simulink model "Torque_Control"  (R2022a)
settings: Solver=FixedStepAuto  StartTime=0.0  StopTime=10.0  RelTol=1e-3
libraries: simulink x9, eeGeneralControl x3
(part 1 of 6)
settings Model: Creator=cspt  LastModifiedBy=joser
settings SolverCC: AlgebraicLoopSolver=TrustRegion
settings DataIOCC: ReturnWorkspaceOutputs=off
settings DebuggingCC: UnconnectedInputMsg=warning  UnconnectedOutputMsg=warning  UnconnectedLineMsg=warning  ArithmeticOperatorsInVariantConditions=warning
settings SFSimCC: SimUseLocalCustomCode=off  CustomCodeUndefinedFunction=UseInterfaceOnly
settings RTWCC: Description=INTECRIO Real-Time Target  SystemTargetFile=irt.tlc  TemplateMakefile=irt_default_tmf  RTWUseLocalCustomCode=off
settings STFCustomTargetCC: TargetLangStandard=C99 (ISO)  UtilityFuncGeneration=Shared location  SystemTargetFile=irt.tlc
settings GRTTargetCC: UtilityFuncGeneration=Shared location  ParMdlRefBuildCompliant=off  CompOptLevelCompliant=off  ConcurrentExecutionCompliant=off  CombineOutputUpdateFcns=off  MatFileLogging=off  CPPClassGenCompliant=off  GRTInterface=on  UseToolchainInfoCompliant=off  GenerateASAP2=on

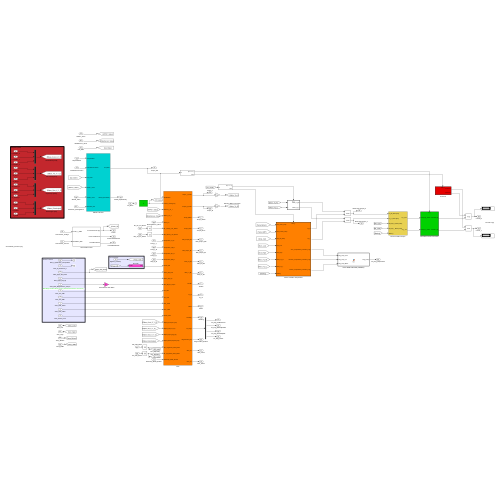
[thumbnail: Simulink's stored preview of the top-level diagram]
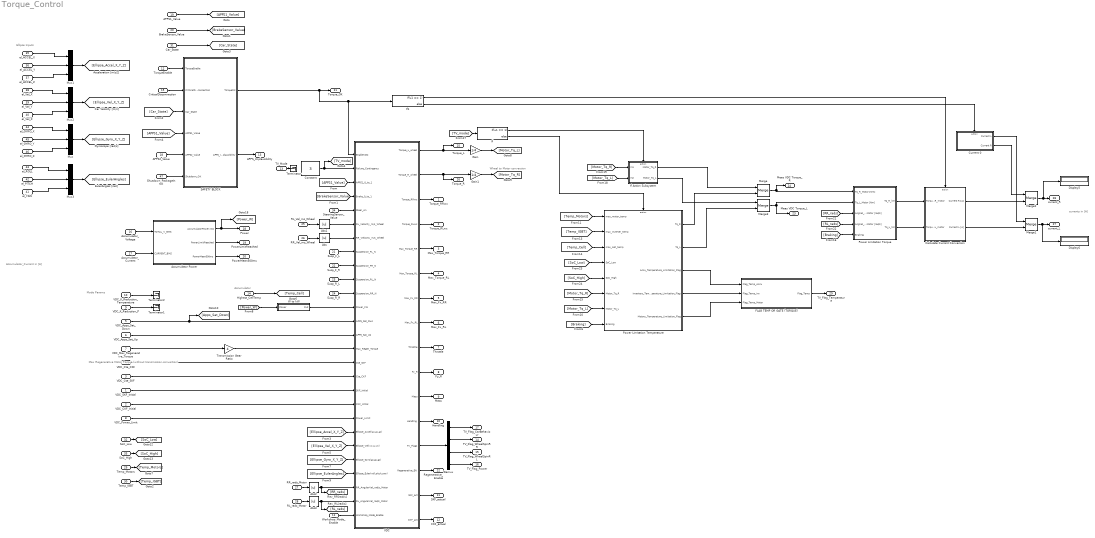
== system Torque_Control ==
  note: Ellipse Inputs
  note: Accumulator_Current in [A]
  note: Wheel to Motor conversion
  note: Max Regenerative Motor Torque (without transmission convertion)
  note: Mode Params
  note: Accumulator
  note: currents in [A]
  VDC_SKF_Initial : Inport
  VDC_CKF_Initial : Inport  Port=2
  VDC_Cte_SKF : Inport  Port=3
  VDC_Cte_CKF : Inport  Port=4
  VDC_Apps_Sat_Down : Inport  Port=5
  VDC_Apps_Sat_Up : Inport  Port=6
  VDC_Max_Regenerative_Torque : Inport  Port=7
  VDC_Power_Limit : Inport  Port=8
  VDC_K_Reduction_P : Inport  Port=9
  VDC_K_Reduction_Temperature : Inport  Port=10
  Workshop_Mode_Enable : Inport  Port=11
  TorqueEnable : Inport  Port=12
  TV_Mode : Inport  Port=13
  Highest_CellTemp : Inport  Port=14
  CriticalDisconnection : Inport  Port=15
  Accumulator_Voltage : Inport  Port=16
  Accumulator_Current : Inport  Port=17
  APPS2_Value : Inport  Port=18
  APPS1_Value : Inport  Port=19
  BrakeSensor_Value : Inport  Port=20
  Susp_F_L : Inport  Port=21
  Susp_F_R : Inport  Port=22
  Susp_R_L : Inport  Port=23
  Susp_R_R : Inport  Port=24
  RL_Vel_ms_Wheel : Inport  Port=25
  RR_Vel_ms_Wheel : Inport  Port=26
  RR_rads_Motor : Inport  Port=27
  RL_rads_Motor : Inport  Port=28
  Temp_Motors : Inport  Port=29
  Temp_IGBT : Inport  Port=30
  Car_State : Inport  Port=31
  SoC_Low : Inport  Port=32
  SoC_High : Inport  Port=33
  SteeringSensor_Value : Inport  Port=34
  el_ACCEL_X : Inport  Port=35
  el_ACCEL_Y : Inport  Port=36
  el_ACCEL_Z : Inport  Port=37
  el_Vel_X : Inport  Port=38
  el_Vel_Y : Inport  Port=39
  el_Vel_Z : Inport  Port=40
  el_YAW : Inport  Port=41
  el_PITCH : Inport  Port=42
  el_ROLL : Inport  Port=43
  el_GYRO_X : Inport  Port=44
  el_GYRO_Y : Inport  Port=45
  el_GYRO_Z : Inport  Port=46
  Shutdown_PackageIntck : Inport  Port=47
  Abs{,1..3} (4 alike) : Abs  SaturateOnIntegerOverflow=off
  Accumulator Power : Subsystem
  Calculate Current Conversion : Subsystem
  Constant : Constant  Value=3
  Current 0 : Subsystem  TreatAsAtomicUnit=on
  Demux : Demux
  Display5 : Display
  Display6 : Display
  FLAG TEMP OR GATE (TORQUE) : MATLAB Function  TreatAsAtomicUnit=on
  Gain : Gain  Gain=1/4
  Gain1 : Gain  Gain=1/4
  If : If  IfExpression=u1 == 1
  If Action Subsystem : Subsystem  TreatAsAtomicUnit=on
  If1 : If  IfExpression=u1 == 1
  Merge{,1..3} (4 alike) : Merge
  Mux{,1..3} (4 alike) : Mux  Inputs=3
  Power Limitation Temperature : Subsystem  TreatAsAtomicUnit=on
  Power Limitation Torque : Subsystem
  SAFETY BLOCK : Subsystem
  Terminator : Terminator
  Terminator1 : Terminator
  Terminator2 : Terminator
  Transmission Gear Ratio : Gain  Gain=4
  VDC : Subsystem
  W to kW : Subsystem
  Torque_RRwc : Outport  VectorParamsAs1DForOutWhenUnconnected=off
  Torque_RLwc : Outport  Port=2  VectorParamsAs1DForOutWhenUnconnected=off
  Max_Torque_RR : Outport  Port=3  VectorParamsAs1DForOutWhenUnconnected=off
  Max_Torque_RL : Outport  Port=4  VectorParamsAs1DForOutWhenUnconnected=off
  Max_Fx_RR : Outport  Port=5  VectorParamsAs1DForOutWhenUnconnected=off
  Max_Fx_RL : Outport  Port=6  VectorParamsAs1DForOutWhenUnconnected=off
  Throttle : Outport  Port=7  VectorParamsAs1DForOutWhenUnconnected=off
  Fy_R : Outport  Port=8  VectorParamsAs1DForOutWhenUnconnected=off
  Mass : Outport  Port=9  VectorParamsAs1DForOutWhenUnconnected=off
  Handling : Outport  Port=10  VectorParamsAs1DForOutWhenUnconnected=off
  SKF_actual : Outport  Port=11  VectorParamsAs1DForOutWhenUnconnected=off
  CKF_actual : Outport  Port=12  VectorParamsAs1DForOutWhenUnconnected=off
  APPS_Implausibility : Outport  Port=13  VectorParamsAs1DForOutWhenUnconnected=off
  TV_Flag_WheelSpinRR : Outport  Port=14  VectorParamsAs1DForOutWhenUnconnected=off
  TV_Flag_WheelSpinRL : Outport  Port=15  VectorParamsAs1DForOutWhenUnconnected=off
  TV_Flag_Power : Outport  Port=16  VectorParamsAs1DForOutWhenUnconnected=off
  TV_Flag_CarBehaviour : Outport  Port=17  VectorParamsAs1DForOutWhenUnconnected=off
  Power : Outport  Port=18  VectorParamsAs1DForOutWhenUnconnected=off
  PowerLimitReached : Outport  Port=19  VectorParamsAs1DForOutWhenUnconnected=off
  PowerMean500ms : Outport  Port=20  VectorParamsAs1DForOutWhenUnconnected=off
  Torque_OK : Outport  Port=21  VectorParamsAs1DForOutWhenUnconnected=off
  Regenerative_Enable : Outport  Port=22  VectorParamsAs1DForOutWhenUnconnected=off
  Meas VDC Torque_L : Outport  Port=23  VectorParamsAs1DForOutWhenUnconnected=off
  Meas VDC Torque_R : Outport  Port=24  VectorParamsAs1DForOutWhenUnconnected=off
  Torque_L : Outport  Port=25  VectorParamsAs1DForOutWhenUnconnected=off
  Torque_R : Outport  Port=26  VectorParamsAs1DForOutWhenUnconnected=off
  current_L : Outport  Port=27  VectorParamsAs1DForOutWhenUnconnected=off
  current_R : Outport  Port=28  VectorParamsAs1DForOutWhenUnconnected=off
  TV_Flag_Temperature : Outport  Port=29  VectorParamsAs1DForOutWhenUnconnected=off
  wires:
  Accumulator Power/1(AccumulatorPower [W]) -> [Power_W], Power/1
  Workshop_Mode_Enable/1 -> VDC/27(Workshop_Mode_Enable)
  SAFETY BLOCK/2(APPS_Implausibility) -> APPS_Implausibility/1
  VDC_Cte_SKF/1 -> VDC/17(Cte_CKF)
  VDC_Apps_Sat_Down/1 -> [Apps_Sat_Down], VDC/13(APPS_Sat_Dwn)
  VDC_Cte_CKF/1 -> VDC/16(Cte_SKF)
  VDC_SKF_Initial/1 -> VDC/18(SKF_Initial)
  VDC/3(Torque_RRwc) -> Torque_RRwc/1
  Highest_CellTemp/1 -> [Temp_Cell]
  [Car_State] -> SAFETY BLOCK/3(Car_State)
  Accumulator_Current/1 -> Accumulator Power/2(CURRENT_BMS)
  Accumulator Power/3(PowerMean500ms) -> PowerMean500ms/1
  Demux/1 -> TV_Flag_CarBehaviour/1
  VDC/14(Regenerative_EN) -> Regenerative_Enable/1
  VDC/10(Fy_R) -> Fy_R/1
  If1/2 -> Current 0/Action
  If1/1 -> Calculate Current Conversion/Action
  TorqueEnable/1 -> SAFETY BLOCK/1(TorqueEnable)
  VDC/5(Max_Torque_RR) -> Max_Torque_RR/1
  Accumulator_Voltage/1 -> Accumulator Power/1(TOTAL_V_BMS)
  Accumulator Power/2(PowerLimitReached) -> PowerLimitReached/1
  VDC/7(Max_Fx_RR) -> Max_Fx_RR/1
  VDC/8(Max_Fx_RL) -> Max_Fx_RL/1
  VDC_CKF_Initial/1 -> VDC/19(CKF_Initial)
  Demux/2 -> TV_Flag_WheelSpinRR/1
  VDC/9(Throttle) -> Throttle/1
  Demux/3 -> TV_Flag_WheelSpinRL/1
  [Power_W] -> W to kW/1(Power)
  CriticalDisconnection/1 -> SAFETY BLOCK/2(CriticalDisconnection)
  VDC/11(Mass) -> Mass/1
  VDC/16(CKF_act) -> CKF_actual/1
  VDC/12(Handling) -> Handling/1
  VDC/13(TV_Flags) -> Demux/1
  VDC/6(Max_Torque_RL) -> Max_Torque_RL/1
  VDC/15(SKF_act) -> SKF_actual/1
  VDC/4(Torque_RLwc) -> Torque_RLwc/1
  APPS1_Value/1 -> [APPS1_Value]
  BrakeSensor_Value/1 -> [BrakeSensor_Value]
  Susp_F_L/1 -> VDC/8(Suspension_FL_N)
  Susp_F_R/1 -> VDC/9(Suspension_FR_N)
  Susp_R_L/1 -> VDC/10(Suspension_RL_N)
  Susp_R_R/1 -> VDC/11(Suspension_RR_N)
  APPS2_Value/1 -> SAFETY BLOCK/5(APPS2_Value)
  Car_State/1 -> [Car_State]
  Abs/1 -> VDC/7(RR_Velocity_m/s_Wheel)
  Abs1/1 -> VDC/6(RL_Velocity_m/s_Wheel)
  Abs2/1 -> [RR_rads], VDC/25(RR_AngularVel_rad/s_Motor)
  Merge1/1 -> current_L/1, Display6/1
  Merge2/1 -> Display5/1, current_R/1
  W to kW/1(Out) -> VDC/12(Power_kW)
  VDC_K_Reduction_P/1 -> Terminator1/1
  VDC_K_Reduction_Temperature/1 -> Terminator2/1
  Demux/4 -> TV_Flag_Power/1
  Current 0/1(Current L) -> Merge1/1
  Transmission Gear Ratio/1 -> VDC/15(Max_Regen_Torque)
  Temp_Motors/1 -> [Temp_Motors]
  Temp_IGBT/1 -> [Temp_IGBT]
  VDC/1(Torque_L_wheel) -> Torque_L/1, Gain/1
  [APPS1_Value] -> VDC/3(APPS1_0_to_1)
  [BrakeSensor_Value] -> VDC/4(Brake_0_to_1)
  [Motor_Tq_R] -> Power Limitation Temperature/6(Motor_Tq_R)
  [Motor_Tq_L] -> Power Limitation Temperature/7(Motor_Tq_L)
  [Temp_Motors] -> Power Limitation Temperature/1(max_motor_temp)
  SoC_High/1 -> [SoC_High]
  [Temp_Cell] -> Power Limitation Temperature/3(max_cell_temp)
  Power Limitation Temperature/4(Inverters_Temperature_Limitation_Flag) -> FLAG TEMP OR GATE (TORQUE)/2(Flag_Temp_Inv)
  Power Limitation Temperature/3(Accu_Temperature_Limitation_Flag) -> FLAG TEMP OR GATE (TORQUE)/1(Flag_Temp_Accu)
  [TV_mode] -> If/1
  Gain1/1 -> [Motor_Tq_R]
  Gain/1 -> [Motor_Tq_L]
  Merge3/1 -> Power Limitation Torque/2(Tq_L_Motor [Nm]), Meas VDC Torque_L/1
  If/1 -> If Action Subsystem/Action
  [Motor_Tq_R] -> If Action Subsystem/1(In1)
  [Motor_Tq_L] -> If Action Subsystem/2(In2)
  Merge/1 -> Power Limitation Torque/1(Tq_R_Motor [Nm]), Meas VDC Torque_R/1
  If/2 -> Power Limitation Temperature/Action
  If Action Subsystem/1(Motor_Tq_R) -> Merge/1
  If Action Subsystem/2(Motor_Tq_L) -> Merge3/1
  Power Limitation Temperature/1(Tq_R) -> Merge/2
  Power Limitation Temperature/2(Tq_L) -> Merge3/2
  RL_Vel_ms_Wheel/1 -> Abs1/1
  RR_Vel_ms_Wheel/1 -> Abs/1
  RR_rads_Motor/1 -> Abs2/1
  RL_rads_Motor/1 -> Abs3/1
  VDC_Max_Regenerative_Torque/1 -> Transmission Gear Ratio/1
  SoC_Low/1 -> [SoC_Low]
  [Temp_IGBT] -> Power Limitation Temperature/2(max_inverter_temp)
  Power Limitation Temperature/5(Motors_Temperature_Limitation_Flag) -> FLAG TEMP OR GATE (TORQUE)/3(Flag_Temp_Motor)
  [Braking] -> Power Limitation Temperature/8(Braking)
  Current 0/2(Current R) -> Merge2/1
  SAFETY BLOCK/1(TorqueOK) -> Torque_OK/1, If1/1, VDC/1(EnableVDC)
  [RR_rads] -> Power Limitation Torque/3(AngVel_R_Motor [rad/s])
  [RL_rads] -> Power Limitation Torque/4(AngVel_L_Motor [rad/s])
  [Braking] -> Power Limitation Torque/5(Braking)
  Power Limitation Torque/1(Tq_R_lim) -> Calculate Current Conversion/1(Torque_R_motor)
  Power Limitation Torque/2(Tq_L_lim) -> Calculate Current Conversion/2(Torque_L_motor)
  TV_Mode/1 -> Terminator/1
  SteeringSensor_Value/1 -> VDC/5(Steer_An)
  [APPS1_Value] -> SAFETY BLOCK/4(APPS1_Value)
  VDC_Power_Limit/1 -> VDC/20(Power_Limit)
  FLAG TEMP OR GATE (TORQUE)/1(Flag_Temp) -> TV_Flag_Temperature/1
  [SoC_High] -> Power Limitation Temperature/5(SoC_High)
  [SoC_Low] -> Power Limitation Temperature/4(SoC_Low)
  Shutdown_PackageIntck/1 -> SAFETY BLOCK/6(Shutdown_OK)
  VDC_Apps_Sat_Up/1 -> VDC/14(APPS_Sat_Up)
  Calculate Current Conversion/1(Current R [A]) -> Merge2/2
  Calculate Current Conversion/2(Current L [A]) -> Merge1/2
  Mux/1 -> [Ellipse_Gyro_X_Y_Z]
  el_Vel_Y/1 -> Mux2/2
  el_GYRO_Z/1 -> Mux/3
  el_Vel_X/1 -> Mux2/1
  el_GYRO_X/1 -> Mux/1
  el_GYRO_Y/1 -> Mux/2
  el_ACCEL_Z/1 -> Mux1/3
  el_ACCEL_Y/1 -> Mux1/2
  Mux2/1 -> [Ellipse_Vel_X_Y_Z]
  el_ACCEL_X/1 -> Mux1/1
  el_Vel_Z/1 -> Mux2/3
  Mux1/1 -> [Ellipse_Accel_X_Y_Z]
  el_YAW/1 -> Mux3/3
  el_PITCH/1 -> Mux3/2
  Mux3/1 -> [Ellipse_EulerAngles]
  el_ROLL/1 -> Mux3/1
  [Ellipse_Accel_X_Y_Z] -> VDC/21(Ellipse_Accel(ax,ay,az))
  [Ellipse_EulerAngles] -> VDC/24(Ellipse_Euler(roll,pitch,yaw))
  [Ellipse_Gyro_X_Y_Z] -> VDC/23(Ellipse_Gyro(gx,gy,gz))
  [Ellipse_Vel_X_Y_Z] -> VDC/22(Ellipse_Vel(vx,vy,vz))
  Constant/1 -> [TV_mode], VDC/2(Failure_Contingency)
  Abs3/1 -> [RL_rads], VDC/26(RL_AngularVel_rad/s_Motor)
  VDC/2(Torque_R_wheel) -> Torque_R/1, Gain1/1

== system Torque_Control/Accumulator Power ==
  TOTAL_V_BMS : Inport
  CURRENT_BMS : Inport  Port=2
  PowerLimitDetection : Subsystem  TreatAsAtomicUnit=on
  Product : Product
  AccumulatorPower [W] : Outport  VectorParamsAs1DForOutWhenUnconnected=off
  PowerLimitReached : Outport  Port=2  VectorParamsAs1DForOutWhenUnconnected=off
  PowerMean500ms : Outport  Port=3  VectorParamsAs1DForOutWhenUnconnected=off
  wires:
  Product/1 -> AccumulatorPower [W]/1, PowerLimitDetection/1(Power)
  PowerLimitDetection/1(PowerLimitReached) -> PowerLimitReached/1
  PowerLimitDetection/2(PowerMean500ms) -> PowerMean500ms/1
  TOTAL_V_BMS/1 -> Product/1
  CURRENT_BMS/1 -> Product/2

== system Torque_Control/Calculate Current Conversion ==
  Torque_R_motor : Inport
  Torque_L_motor : Inport  Port=2
  Action Port : ActionPort  ActionPortLabel=if { }
  Gain : Gain  Gain=-1
  KT_L_TORKY : Subsystem  TreatAsAtomicUnit=on
  KT_R_EMY : Subsystem  TreatAsAtomicUnit=on
  Current R [A] : Outport  VectorParamsAs1DForOutWhenUnconnected=off
  Current L [A] : Outport  Port=2  VectorParamsAs1DForOutWhenUnconnected=off
  wires:
  Torque_R_motor/1 -> KT_R_EMY/1(Torque)
  Torque_L_motor/1 -> KT_L_TORKY/1(Torque)
  Gain/1 -> Current L [A]/1
  KT_R_EMY/1(Current) -> Current R [A]/1
  KT_L_TORKY/1(Current) -> Gain/1

== system Torque_Control/Current 0 ==
  Action Port : ActionPort  ActionPortLabel=else { }
  Constant : Constant  Value=0
  Current L : Outport  VectorParamsAs1DForOutWhenUnconnected=off
  Current R : Outport  Port=2  VectorParamsAs1DForOutWhenUnconnected=off
  wires:
  Constant/1 -> Current R/1, Current L/1

== system Torque_Control/If Action Subsystem ==
  note: Tq already limited (because of Temp and Power) with the SoC
  In1 : Inport
  In2 : Inport  Port=2
  Action Port : ActionPort  ActionPortLabel=if { }
  Motor_Tq_R : Outport  VectorParamsAs1DForOutWhenUnconnected=off
  Motor_Tq_L : Outport  Port=2  VectorParamsAs1DForOutWhenUnconnected=off
  wires:
  In1/1 -> Motor_Tq_R/1
  In2/1 -> Motor_Tq_L/1

== system Torque_Control/Power Limitation Temperature ==
  note: Outputs:
      | Flags: 1 means power is being limited by temperature, 0 means not limited
      | SoP_discharge: State of Power for discharging
      | SoP_charge: State of Power for charging
  note: Inputs:
      | max_cell_temp: signal from AMS_Master (Highest_Cell_Temp) [ºC]
      | max_inverter_temp: highest temperature of any of the inverters [ºC]
      | max_motor_temp: highest temperature of any of the motors [ºC]
      | SoC_Low, SoC_High: Lowest & Highest cell state of charge (0-100) [%]
  max_motor_temp : Inport
  max_inverter_temp : Inport  Port=2
  max_cell_temp : Inport  Port=3
  SoC_Low : Inport  Port=4
  SoC_High : Inport  Port=5
  Motor_Tq_R : Inport  Port=6
  Motor_Tq_L : Inport  Port=7
  Braking : Inport  Port=8
  Action Port : ActionPort  ActionPortLabel=else { }
  Max_Tq_per_motor : Constant  Value=120
  Saturation : Saturate  UpperLimit=1  LowerLimit=0
  Saturation1 : Saturate  UpperLimit=1  LowerLimit=0
  SoC_SoP : Subsystem
  Torque Limitation Temperature Controller : MATLAB Function  TreatAsAtomicUnit=on
  initial_limitation : Constant  Value=0.4
  temperature_SoP : Subsystem
  Tq_R : Outport  VectorParamsAs1DForOutWhenUnconnected=off
  Tq_L : Outport  Port=2  VectorParamsAs1DForOutWhenUnconnected=off
  Accu_Temperature_Limitation_Flag : Outport  Port=3
  Inverters_Temperature_Limitation_Flag : Outport  Port=4
  Motors_Temperature_Limitation_Flag : Outport  Port=5
  wires:
  temperature_SoP/1(SoP) -> SoC_SoP/3(SoP_Temperature)  "temperature_SoP"
  SoC_Low/1 -> SoC_SoP/1(SoC_Low)
  Saturation1/1 -> Torque Limitation Temperature Controller/2(SoP_Charge)
  SoC_High/1 -> SoC_SoP/2(SoC_High)
  initial_limitation/1 -> temperature_SoP/4(initial_limitation)
  Saturation/1 -> Torque Limitation Temperature Controller/1(SoP_Discharge)
  temperature_SoP/4(Motors_Temperature_Limitation_Flag) -> Motors_Temperature_Limitation_Flag/1
  temperature_SoP/2(Accu_Temperature_Limitation_Flag) -> Accu_Temperature_Limitation_Flag/1
  SoC_SoP/2(SoP_Regen) -> Saturation1/1  "SoP_Regen"
  max_inverter_temp/1 -> temperature_SoP/2(max_inverter_temp)
  SoC_SoP/1(SoP_Discharge) -> Saturation/1  "SoP_Discharge"
  temperature_SoP/3(Inverters_Temperature_Limitation_Flag) -> Inverters_Temperature_Limitation_Flag/1
  max_cell_temp/1 -> temperature_SoP/3(max_cell_temp), SoC_SoP/4(max_cell_temp)
  max_motor_temp/1 -> temperature_SoP/1(max_motor_temp)
  Braking/1 -> Torque Limitation Temperature Controller/3(Braking)
  Motor_Tq_R/1 -> Torque Limitation Temperature Controller/4(Tq_R)
  Motor_Tq_L/1 -> Torque Limitation Temperature Controller/5(Tq_L)
  Torque Limitation Temperature Controller/1(Tq_R_limited) -> Tq_R/1
  Torque Limitation Temperature Controller/2(Tq_L_limited) -> Tq_L/1
  Max_Tq_per_motor/1 -> Torque Limitation Temperature Controller/6(Max_Tq_per_motor)

== system Torque_Control/Power Limitation Torque ==
  Tq_R_Motor [Nm] : Inport
  Tq_L_Motor [Nm] : Inport  Port=2
  AngVel_R_Motor [rad/s] : Inport  Port=3
  AngVel_L_Motor [rad/s] : Inport  Port=4
  Braking : Inport  Port=5
  MATLAB Function : MATLAB Function  TreatAsAtomicUnit=on
  Max_Power_charge [kW] : Constant  Value=60
  Max_Power_discharge [kW] : Constant  Value=80
  Tq_R_lim : Outport  VectorParamsAs1DForOutWhenUnconnected=off
  Tq_L_lim : Outport  Port=2  VectorParamsAs1DForOutWhenUnconnected=off
  wires:
  Tq_R_Motor [Nm]/1 -> MATLAB Function/1(Tq_R)
  Tq_L_Motor [Nm]/1 -> MATLAB Function/2(Tq_L)
  AngVel_R_Motor [rad/s]/1 -> MATLAB Function/3(AngVel_R)
  AngVel_L_Motor [rad/s]/1 -> MATLAB Function/4(AngVel_L)
  Braking/1 -> MATLAB Function/5(Braking)
  Max_Power_discharge [kW]/1 -> MATLAB Function/6(Max_Power_Discharge)
  Max_Power_charge [kW]/1 -> MATLAB Function/7(Max_Power_Charge)
  MATLAB Function/1(Tq_R_lim) -> Tq_R_lim/1
  MATLAB Function/2(Tq_L_lim) -> Tq_L_lim/1

== system Torque_Control/SAFETY BLOCK ==
  note: CriticalDisconnection -> 1
      | OK -> 0
  note: Opened -> 0
      | OK -> 1
  TorqueEnable : Inport
  CriticalDisconnection : Inport  Port=2
  Car_State : Inport  Port=3
  APPS1_Value : Inport  Port=4
  APPS2_Value : Inport  Port=5
  Shutdown_OK : Inport  Port=6
  APPS_IMPLAUSIBILITY : Subsystem
  Compare To Constant : simulink/Logic and Bit Operations/Compare To Constant  relop===  const=15  OutDataTypeStr=boolean
  Logical Operator : Logic  Inputs=5  OutDataTypeStr=boolean
  Logical Operator1 : Logic  Operator=NOT  IconShape=distinctive  AllPortsSameDT=off  OutDataTypeStr=boolean
  NOT : Logic  Operator=NOT  IconShape=distinctive  AllPortsSameDT=off  OutDataTypeStr=boolean
  TorqueOK : Outport  VectorParamsAs1DForOutWhenUnconnected=off
  APPS_Implausibility : Outport  Port=2  VectorParamsAs1DForOutWhenUnconnected=off
  wires:
  Logical Operator/1 -> TorqueOK/1
  Car_State/1 -> Compare To Constant/1
  NOT/1 -> Logical Operator/3
  CriticalDisconnection/1 -> NOT/1
  TorqueEnable/1 -> Logical Operator/2
  APPS2_Value/1 -> APPS_IMPLAUSIBILITY/2(APPS2)
  APPS1_Value/1 -> APPS_IMPLAUSIBILITY/1(APPS1)
  Logical Operator1/1 -> APPS_Implausibility/1
  Compare To Constant/1 -> Logical Operator/4
  APPS_IMPLAUSIBILITY/1(OK) -> Logical Operator/5, Logical Operator1/1
  Shutdown_OK/1 -> Logical Operator/1

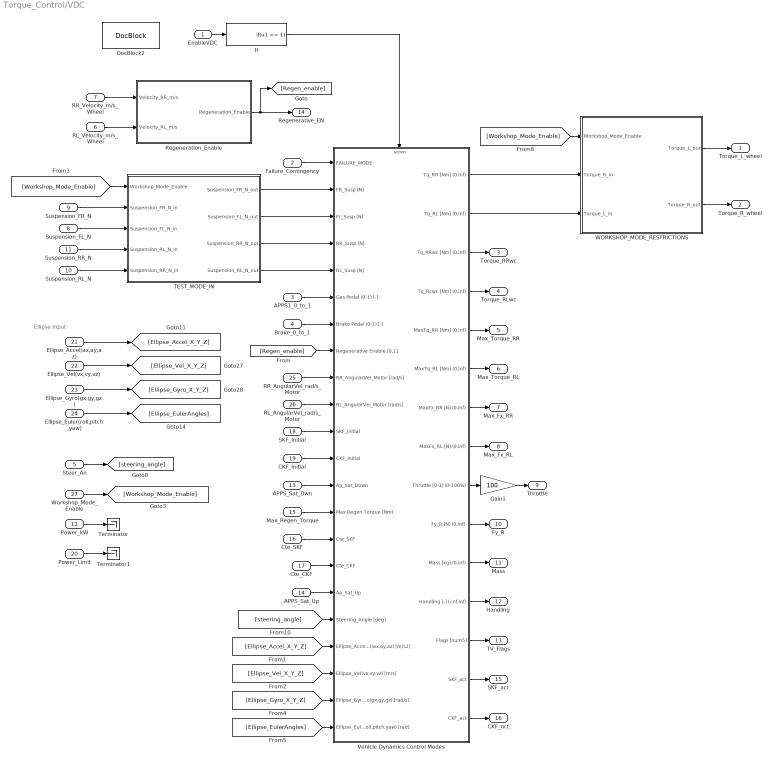
== system Torque_Control/VDC ==
  note: Ellipse Input
  EnableVDC : Inport
  Failure_Contingency : Inport  Port=2
  APPS1_0_to_1 : Inport  Port=3
  Brake_0_to_1 : Inport  Port=4
  Steer_An : Inport  Port=5
  RL_Velocity_m/s_Wheel : Inport  Port=6
  RR_Velocity_m/s_Wheel : Inport  Port=7
  Suspension_FL_N : Inport  Port=8
  Suspension_FR_N : Inport  Port=9
  Suspension_RL_N : Inport  Port=10
  Suspension_RR_N : Inport  Port=11
  Power_kW : Inport  Port=12
  APPS_Sat_Dwn : Inport  Port=13
  APPS_Sat_Up : Inport  Port=14
  Max_Regen_Torque : Inport  Port=15
  Cte_SKF : Inport  Port=16
  Cte_CKF : Inport  Port=17
  SKF_Initial : Inport  Port=18
  CKF_Initial : Inport  Port=19
  Power_Limit : Inport  Port=20
  Ellipse_Accel(ax,ay,az) : Inport  Port=21
  Ellipse_Vel(vx,vy,vz) : Inport  Port=22
  Ellipse_Gyro(gx,gy,gz) : Inport  Port=23
  Ellipse_Euler(roll,pitch,yaw) : Inport  Port=24
  RR_AngularVel_rad/s_Motor : Inport  Port=25
  RL_AngularVel_rad/s_Motor : Inport  Port=26
  Workshop_Mode_Enable : Inport  Port=27
  DocBlock2 : simulink/Model-Wide Utilities/DocBlock  DocumentType=Text
      content=|
      | Enable Vehicle Dynamics Control.
      |
      | This port must be 1 if the calculations for VDC must be made
  Gain1 : Gain  Gain=100
  If : If  IfExpression=u1 == 1  ShowElse=off
  Regeneration_Enable : Subsystem  TreatAsAtomicUnit=on
  TEST_MODE_IN : Subsystem  TreatAsAtomicUnit=on
  Terminator : Terminator
  Terminator1 : Terminator
  Vehicle Dynamics Control Modes : Subsystem
  WORKSHOP_MODE_RESTRICTIONS : Subsystem  TreatAsAtomicUnit=on
  Torque_L_wheel : Outport  VectorParamsAs1DForOutWhenUnconnected=off
  Torque_R_wheel : Outport  Port=2  VectorParamsAs1DForOutWhenUnconnected=off
  Torque_RRwc : Outport  Port=3  VectorParamsAs1DForOutWhenUnconnected=off
  Torque_RLwc : Outport  Port=4  VectorParamsAs1DForOutWhenUnconnected=off
  Max_Torque_RR : Outport  Port=5  VectorParamsAs1DForOutWhenUnconnected=off
  Max_Torque_RL : Outport  Port=6  VectorParamsAs1DForOutWhenUnconnected=off
  Max_Fx_RR : Outport  Port=7  VectorParamsAs1DForOutWhenUnconnected=off
  Max_Fx_RL : Outport  Port=8  VectorParamsAs1DForOutWhenUnconnected=off
  Throttle : Outport  Port=9  VectorParamsAs1DForOutWhenUnconnected=off
  Fy_R : Outport  Port=10  VectorParamsAs1DForOutWhenUnconnected=off
  Mass : Outport  Port=11  VectorParamsAs1DForOutWhenUnconnected=off
  Handling : Outport  Port=12  VectorParamsAs1DForOutWhenUnconnected=off
  TV_Flags : Outport  Port=13  VectorParamsAs1DForOutWhenUnconnected=off
  Regenerative_EN : Outport  Port=14  VectorParamsAs1DForOutWhenUnconnected=off
  SKF_act : Outport  Port=15  VectorParamsAs1DForOutWhenUnconnected=off
  CKF_act : Outport  Port=16  VectorParamsAs1DForOutWhenUnconnected=off
  wires:
  RR_Velocity_m/s_Wheel/1 -> Regeneration_Enable/1(Velocity_RR_m/s)
  Gain1/1 -> Throttle/1
  Vehicle Dynamics Control Modes/7(MaxFx_RR [N] (0,inf)) -> Max_Fx_RR/1
  Vehicle Dynamics Control Modes/6(MaxTq_RL [Nm] (0,inf)) -> Max_Torque_RL/1
  Vehicle Dynamics Control Modes/8(MaxFx_RL [N] (0,inf)) -> Max_Fx_RL/1
  Power_kW/1 -> Terminator/1
  Vehicle Dynamics Control Modes/1(Tq_RR [Nm] (0,inf)) -> WORKSHOP_MODE_RESTRICTIONS/2(Torque_R_in)
  APPS_Sat_Up/1 -> Vehicle Dynamics Control Modes/17(Ap_Sat_Up)
  WORKSHOP_MODE_RESTRICTIONS/1(Torque_L_out) -> Torque_L_wheel/1
  Vehicle Dynamics Control Modes/3(Tq_RRwc [Nm] (0,inf)) -> Torque_RRwc/1
  Suspension_FL_N/1 -> TEST_MODE_IN/3(Suspension_FL_N_in)
  Suspension_FR_N/1 -> TEST_MODE_IN/2(Suspension_FR_N_in)
  TEST_MODE_IN/1(Suspension_FR_N_out) -> Vehicle Dynamics Control Modes/2(FR_Susp [N])
  RR_AngularVel_rad/s_Motor/1 -> Vehicle Dynamics Control Modes/9(RR_AngularVel_Motor [rad/s])
  Vehicle Dynamics Control Modes/14(SKF_act) -> SKF_act/1
  APPS1_0_to_1/1 -> Vehicle Dynamics Control Modes/6(Gas Pedal (0-1) [-])
  Vehicle Dynamics Control Modes/4(Tq_RLwc [Nm] (0,inf)) -> Torque_RLwc/1
  Vehicle Dynamics Control Modes/5(MaxTq_RR [Nm] (0,inf)) -> Max_Torque_RR/1
  Brake_0_to_1/1 -> Vehicle Dynamics Control Modes/7(Brake Pedal (0-1) [-])
  RL_Velocity_m/s_Wheel/1 -> Regeneration_Enable/2(Velocity_RL_m/s)
  Vehicle Dynamics Control Modes/11(Mass [kg] (0,inf)) -> Mass/1
  Vehicle Dynamics Control Modes/9(Throttle [0-1] (0-100%)) -> Gain1/1
  Vehicle Dynamics Control Modes/2(Tq_RL [Nm] (0,inf)) -> WORKSHOP_MODE_RESTRICTIONS/3(Torque_L_in)
  EnableVDC/1 -> If/1
  Suspension_RL_N/1 -> TEST_MODE_IN/5(Suspension_RR_N_in)
  Vehicle Dynamics Control Modes/10(Fy_R [N] (0,inf)) -> Fy_R/1
  Vehicle Dynamics Control Modes/13(Flags [num5]) -> TV_Flags/1
  [Workshop_Mode_Enable] -> TEST_MODE_IN/1(Workshop_Mode_Enable)
  Suspension_RR_N/1 -> TEST_MODE_IN/4(Suspension_RL_N_in)
  Vehicle Dynamics Control Modes/12(Handling [-] (-inf,inf)) -> Handling/1
  Workshop_Mode_Enable/1 -> [Workshop_Mode_Enable]
  Vehicle Dynamics Control Modes/15(CKF_act) -> CKF_act/1
  If/1 -> Vehicle Dynamics Control Modes/Action
  TEST_MODE_IN/2(Suspension_FL_N_out) -> Vehicle Dynamics Control Modes/3(FL_Susp [N])
  TEST_MODE_IN/3(Suspension_RR_N_out) -> Vehicle Dynamics Control Modes/4(RR_Susp [N])
  TEST_MODE_IN/4(Suspension_RL_N_out) -> Vehicle Dynamics Control Modes/5(RL_Susp [N])
  RL_AngularVel_rad/s_Motor/1 -> Vehicle Dynamics Control Modes/10(RL_AngularVel_Motor [rad/s])
  SKF_Initial/1 -> Vehicle Dynamics Control Modes/11(SKF_Initial)
  CKF_Initial/1 -> Vehicle Dynamics Control Modes/12(CKF_Initial)
  APPS_Sat_Dwn/1 -> Vehicle Dynamics Control Modes/13(Ap_Sat_Down)
  Max_Regen_Torque/1 -> Vehicle Dynamics Control Modes/14(Max Regen Torque [Nm])
  Cte_SKF/1 -> Vehicle Dynamics Control Modes/15(Cte_SKF)
  Cte_CKF/1 -> Vehicle Dynamics Control Modes/16(Cte_CKF)
  Failure_Contingency/1 -> Vehicle Dynamics Control Modes/1(FAILURE_MODE)
  [Regen_enable] -> Vehicle Dynamics Control Modes/8(Regenerative Enable [0,1])
  WORKSHOP_MODE_RESTRICTIONS/2(Torque_R_out) -> Torque_R_wheel/1
  [Workshop_Mode_Enable] -> WORKSHOP_MODE_RESTRICTIONS/1(Workshop_Mode_Enable)
  Regeneration_Enable/1(Regeneration_Enable) -> Regenerative_EN/1, [Regen_enable]
  Steer_An/1 -> [steering_angle]
  [steering_angle] -> Vehicle Dynamics Control Modes/18(Steering_Angle [deg])
  Power_Limit/1 -> Terminator1/1
  Ellipse_Euler(roll,pitch,yaw)/1 -> [Ellipse_EulerAngles]
  Ellipse_Gyro(gx,gy,gz)/1 -> [Ellipse_Gyro_X_Y_Z]
  Ellipse_Vel(vx,vy,vz)/1 -> [Ellipse_Vel_X_Y_Z]
  Ellipse_Accel(ax,ay,az)/1 -> [Ellipse_Accel_X_Y_Z]
  [Ellipse_EulerAngles] -> Vehicle Dynamics Control Modes/22(Ellipse_Euler(roll,pitch,yaw) [rad])
  [Ellipse_Gyro_X_Y_Z] -> Vehicle Dynamics Control Modes/21(Ellipse_Gyro(gx,gy,gz) [rad/s])
  [Ellipse_Vel_X_Y_Z] -> Vehicle Dynamics Control Modes/20(Ellipse_Vel(vx,vy,vz) [m/s])
  [Ellipse_Accel_X_Y_Z] -> Vehicle Dynamics Control Modes/19(Ellipse_Accel(ax,ay,az) [m/s2])

== system Torque_Control/W to kW ==
  Power : Inport
  0-100 to 0-2 : Constant  Value=1000
  Divide5 : Product  Inputs=*/
  Out : Outport  VectorParamsAs1DForOutWhenUnconnected=off
  wires:
  Power/1 -> Divide5/1
  0-100 to 0-2/1 -> Divide5/2
  Divide5/1 -> Out/1

== system Torque_Control/Accumulator Power/PowerLimitDetection ==
  note: mean:500ms
      | time:25ms
      | moving window: 500/25=20
  Power : Inport
  Data Store Memory10 : DataStoreMemory  ReadBeforeWriteMsg=warning  WriteAfterWriteMsg=warning  WriteAfterReadMsg=warning  ShowAdditionalParam=off
  Data Store Read30 : DataStoreRead  IndexOptions=Index vector (dialog)  Indices=1  OutputSizes=1
  Data Store Write20 : DataStoreWrite  IndexOptions=Index vector (dialog)  Indices=1  OutputSizes=1
  If : If  IfExpression=u1 >= 80000
  LimitReached : Subsystem  TreatAsAtomicUnit=on
  Merge1 : Merge
  OK_OrLatch : Subsystem  TreatAsAtomicUnit=on
  PowerLimitReached : Outport  VectorParamsAs1DForOutWhenUnconnected=off
  PowerMean500ms : Outport  Port=2  VectorParamsAs1DForOutWhenUnconnected=off
  wires:
  Power/1 -> If/1, PowerMean500ms/1
  If/1 -> LimitReached/Action
  If/2 -> OK_OrLatch/Action
  LimitReached/1("Out ") -> Merge1/1
  OK_OrLatch/1(Out 1) -> Merge1/2
  Merge1/1 -> Data Store Write20/1, PowerLimitReached/1
  Data Store Read30/1 -> OK_OrLatch/1(IN)

== system Torque_Control/Calculate Current Conversion/KT_L_TORKY ==
  Torque : Inport
  A/Nm : Gain  Gain=0.2
  Current : Outport  VectorParamsAs1DForOutWhenUnconnected=off
  wires:
  A/Nm/1 -> Current/1
  Torque/1 -> A/Nm/1

== system Torque_Control/Calculate Current Conversion/KT_R_EMY ==
  Torque : Inport
  A/Nm : Gain  Gain=0.2
  Current : Outport  VectorParamsAs1DForOutWhenUnconnected=off
  wires:
  Torque/1 -> A/Nm/1
  A/Nm/1 -> Current/1

== system Torque_Control/Power Limitation Temperature/SoC_SoP ==
  note: El lookup se puede obtener ensayando una celda en una descarga y en una carga con pérdidas de calor constantes. La corriente normalizada será el lookup.
  note: Si está descargada, no descargues más
  note: Si está cargada, no
      | cargues más
  SoC_Low : Inport
  SoC_High : Inport  Port=2
  SoP_Temperature : Inport  Port=3
  max_cell_temp : Inport  Port=4
  Gain5 : Gain  Gain=1/100
  Gain6 : Gain  Gain=1/100
  Lookup_SoC_SoP_chg : Lookup_n-D  NumberOfTableDimensions=1  BreakpointsForDimension1=[0.02 0.1 0.2 0.3 0.5 0.8 0.95 1]  Table=[0.95 1 1 1 1 0.9 0.75 0.02]  InternalRulePriority=Speed  RndMeth=Simplest
  Lookup_SoC_SoP_dischg : Lookup_n-D  NumberOfTableDimensions=1  BreakpointsForDimension1=[0.02 0.1 0.2 0.3 0.5 0.8 0.9 1]  Table=[0.4 0.6 0.8 0.95 1 1 0.98 0.95]  InternalRulePriority=Speed  RndMeth=Simplest
  Lookup_Temp_SoP_chg : Lookup_n-D  NumberOfTableDimensions=1  BreakpointsForDimension1=[45 48 49 50 51]  Table=[1 0.75 0.5 0 0]  InternalRulePriority=Speed  RndMeth=Simplest
  Product : Product
  Product4 : Product
  Product5 : Product
  SoP_Discharge : Outport
  SoP_Regen : Outport  Port=2
  wires:
  Lookup_SoC_SoP_dischg/1 -> Product4/1
  Product/1 -> Product5/2
  SoP_Temperature/1 -> Product4/2, Product5/1
  SoC_Low/1 -> Gain6/1
  Gain6/1 -> Lookup_SoC_SoP_dischg/1
  SoC_High/1 -> Gain5/1
  Gain5/1 -> Lookup_SoC_SoP_chg/1
  Product5/1 -> SoP_Regen/1
  Product4/1 -> SoP_Discharge/1
  Lookup_SoC_SoP_chg/1 -> Product/1
  max_cell_temp/1 -> Lookup_Temp_SoP_chg/1
  Lookup_Temp_SoP_chg/1 -> Product/2

== system Torque_Control/Power Limitation Temperature/temperature_SoP ==
  max_motor_temp : Inport
  max_inverter_temp : Inport  Port=2
  max_cell_temp : Inport  Port=3
  initial_limitation : Inport  Port=4
  Flag_Accu : simulink/Logic and Bit Operations/Compare To Constant  relop=<  const=1  OutDataTypeStr=boolean  ZeroCross=off
  Flag_Inv : simulink/Logic and Bit Operations/Compare To Constant  relop=<  const=1  OutDataTypeStr=boolean  ZeroCross=off
  Flag_Mot : simulink/Logic and Bit Operations/Compare To Constant  relop=<  const=1  OutDataTypeStr=boolean  ZeroCross=off
  Min : MinMax  Inputs=3
  temperature_rise_limitator_Accu : Subsystem
  temperature_rise_limitator_Inverters : Subsystem
  temperature_rise_limitator_Motors : Subsystem
  SoP : Outport
  Accu_Temperature_Limitation_Flag : Outport  Port=2
  Inverters_Temperature_Limitation_Flag : Outport  Port=3
  Motors_Temperature_Limitation_Flag : Outport  Port=4
  wires:
  temperature_rise_limitator_Inverters/1(SoP) -> Flag_Inv/1, Min/2
  initial_limitation/1 -> temperature_rise_limitator_Accu/2(initial_limitation), temperature_rise_limitator_Motors/2(initial_limitation), temperature_rise_limitator_Inverters/2(initial_limitation)
  Flag_Accu/1 -> Accu_Temperature_Limitation_Flag/1
  temperature_rise_limitator_Motors/1(SoP) -> Flag_Mot/1, Min/3
  max_cell_temp/1 -> temperature_rise_limitator_Accu/1(max_cell_temp)
  temperature_rise_limitator_Accu/1(SoP) -> Flag_Accu/1, Min/1
  Min/1 -> SoP/1
  Flag_Inv/1 -> Inverters_Temperature_Limitation_Flag/1
  Flag_Mot/1 -> Motors_Temperature_Limitation_Flag/1
  max_inverter_temp/1 -> temperature_rise_limitator_Inverters/1(max_inverter_temp)
  max_motor_temp/1 -> temperature_rise_limitator_Motors/1(max_motor_temp)

== system Torque_Control/SAFETY BLOCK/APPS_IMPLAUSIBILITY ==
  APPS1 : Inport
  APPS2 : Inport  Port=2
  Ab : Abs  SaturateOnIntegerOverflow=off
  If : If  IfExpression=u1 > 0.1
  Imp : Subsystem  TreatAsAtomicUnit=on
  Merge : Merge
  Not Imp : Subsystem  TreatAsAtomicUnit=on
  Sum : Sum  Inputs=|+-
  OK : Outport  VectorParamsAs1DForOutWhenUnconnected=off
  wires:
  APPS1/1 -> Sum/1
  APPS2/1 -> Sum/2
  Sum/1 -> Ab/1
  Ab/1 -> If/1
  Imp/1(Out1) -> Merge/1  "Bool 0"
  Not Imp/1(Out1) -> Merge/2  "Bool 1"
  Merge/1 -> OK/1
  If/2 -> Not Imp/Action
  If/1 -> Imp/Action

== system Torque_Control/VDC/Regeneration_Enable ==
  note: Regen is Enable if velocity is higher than 2 km/h, to avoid backwards velocity due to Regen Tq (negative)
  Velocity_RR_m/s : Inport
  Velocity_RL_m/s : Inport  Port=2
  Enabled : Constant
  "Enabled " : Subsystem  TreatAsAtomicUnit=on
  Gain : Gain  Gain=3.6
  Gain1 : Gain  Gain=3.6
  If : If  NumInputs=2  IfExpression=(u1>2)&(u2>2)
  Merge1 : Merge
  NotEnabled : Subsystem  TreatAsAtomicUnit=on
  "Zero " : Constant  Value=0
  Regeneration_Enable : Outport  VectorParamsAs1DForOutWhenUnconnected=off
  wires:
  Merge1/1 -> Regeneration_Enable/1
  Velocity_RR_m/s/1 -> Gain/1
  Velocity_RL_m/s/1 -> Gain1/1
  If/1 -> "Enabled "/Action
  If/2 -> NotEnabled/Action
  "Zero "/1 -> NotEnabled/1(In1)
  NotEnabled/1(Out1) -> Merge1/2
  "Enabled "/1(Out1) -> Merge1/1
  Enabled/1 -> "Enabled "/1(In1)
  Gain1/1 -> If/2
  Gain/1 -> If/1

== system Torque_Control/VDC/TEST_MODE_IN ==
  Workshop_Mode_Enable : Inport
  Suspension_FR_N_in : Inport  Port=2
  Suspension_FL_N_in : Inport  Port=3
  Suspension_RL_N_in : Inport  Port=4
  Suspension_RR_N_in : Inport  Port=5
  BYPASS : Subsystem  TreatAsAtomicUnit=on
  If : If  IfExpression=u1 == 1
  Merge{,1..3} (4 alike) : Merge
  TEST_CONSTANTS : Subsystem  TreatAsAtomicUnit=on
  Suspension_FR_N_out : Outport  VectorParamsAs1DForOutWhenUnconnected=off
  Suspension_FL_N_out : Outport  Port=2  VectorParamsAs1DForOutWhenUnconnected=off
  Suspension_RR_N_out : Outport  Port=3  VectorParamsAs1DForOutWhenUnconnected=off
  Suspension_RL_N_out : Outport  Port=4  VectorParamsAs1DForOutWhenUnconnected=off
  wires:
  Suspension_FR_N_in/1 -> BYPASS/1(In1)
  Suspension_FL_N_in/1 -> BYPASS/2(In2)
  Suspension_RR_N_in/1 -> BYPASS/3(In3)
  Suspension_RL_N_in/1 -> BYPASS/4(In4)
  Merge/1 -> Suspension_FR_N_out/1
  Merge1/1 -> Suspension_FL_N_out/1
  Merge2/1 -> Suspension_RR_N_out/1
  Merge3/1 -> Suspension_RL_N_out/1
  BYPASS/1(Out1) -> Merge/1
  BYPASS/2(Out2) -> Merge1/1
  BYPASS/3(Out3) -> Merge2/1
  BYPASS/4(Out4) -> Merge3/1
  Workshop_Mode_Enable/1 -> If/1
  If/2 -> BYPASS/Action
  If/1 -> TEST_CONSTANTS/Action
  TEST_CONSTANTS/4(Out4) -> Merge3/2
  TEST_CONSTANTS/3(Out3) -> Merge2/2
  TEST_CONSTANTS/2(Out2) -> Merge1/2
  TEST_CONSTANTS/1(Out1) -> Merge/2

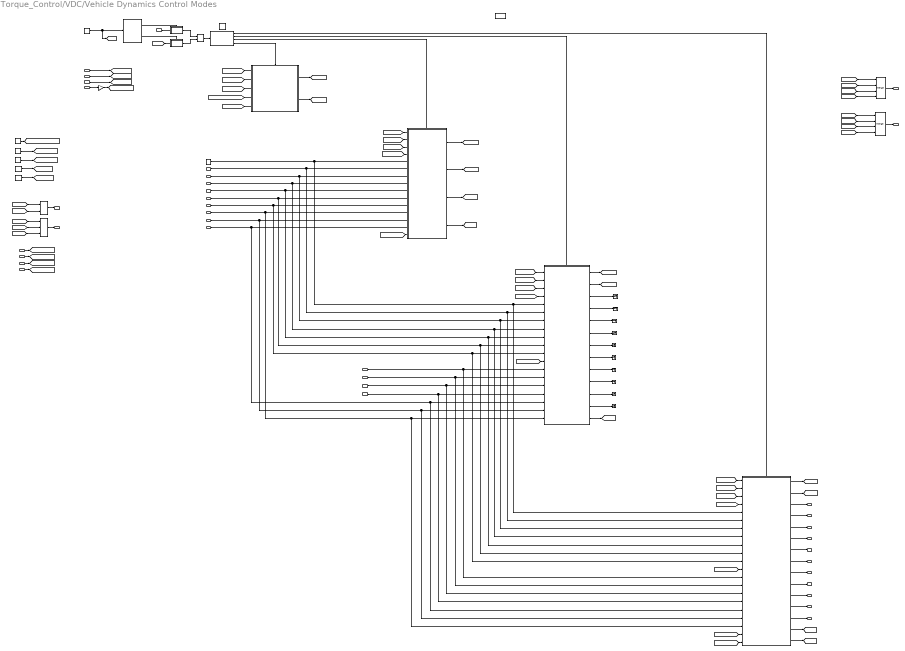
== system Torque_Control/VDC/Vehicle Dynamics Control Modes ==
  note: Handling now is negligible is always 0
  note: Failure Mode Selection: 5 -> Automatic Failure Mode Selection according to sensors available
      | 4 -> Rigid Axle (red)
      | 3 -> Steering TV with TC (orange)
      | 2 -> VDC without longitudinal (yellow)
      | 1 -> VDC complete (green)
      | 0 -> TV with TC 2023
  note: Car constants
  note: Ellipse Inputs
  FAILURE_MODE : Inport
  FR_Susp [N] : Inport  Port=2
  FL_Susp [N] : Inport  Port=3
  RR_Susp [N] : Inport  Port=4
  RL_Susp [N] : Inport  Port=5
  Gas Pedal (0-1) [-] : Inport  Port=6
  Brake Pedal (0-1) [-] : Inport  Port=7
  Regenerative Enable [0,1] : Inport  Port=8
  RR_AngularVel_Motor [rad/s] : Inport  Port=9
  RL_AngularVel_Motor [rad/s] : Inport  Port=10
  SKF_Initial : Inport  Port=11
  CKF_Initial : Inport  Port=12
  Ap_Sat_Down : Inport  Port=13
  Max Regen Torque [Nm] : Inport  Port=14
  Cte_SKF : Inport  Port=15
  Cte_CKF : Inport  Port=16
  Ap_Sat_Up : Inport  Port=17
  Steering_Angle [deg] : Inport  Port=18
  Ellipse_Accel(ax,ay,az) [m/s2] : Inport  Port=19
  Ellipse_Vel(vx,vy,vz) [m/s] : Inport  Port=20
  Ellipse_Gyro(gx,gy,gz) [rad/s] : Inport  Port=21
  Ellipse_Euler(roll,pitch,yaw) [rad] : Inport  Port=22
  Action Port : ActionPort  ActionPortLabel=if { }
  Automatic Failure Mode : Subsystem  TreatAsAtomicUnit=on
  Constant : Constant  Value=5
  DocBlock : simulink/Model-Wide Utilities/DocBlock  DocumentType=Text
      content=|
      | This port activates the different modes that the VDC must be in according
      | to the signals that the Main ECU has available.
      |
      | Port Must be 1 to activate VDC 2018 Complete (Green)
      | Requirement: All sensors are connected (Ellipse, Steering, SuspensionRear
      | [SuspensionFront only needed to calculate Mass]).
      |
      | Port Must be 2 to activate VDC without Longitudinal (Yellow)
      | Requirement: No steering sensor data
      |
      | Port Must be 3 to activate Steering TV 2017 without TC (Orange)
      | Requirement: (No Ellipse) or (No SuspensionRear Data)
      |
      | Port Must be 4 to activate Rigid Axle (Red)
      | Requirement: (No Steering Sensor) and (No Ellipse or No SuspensionRear)
  FAILURE MODE : If  IfExpression=u1 == 1  ElseIfExpressions=u1 == 2, u1 == 3, u1 == 4  ShowElse=off
  Gain : Gain  Gain=-1
  If : If  IfExpression=u1 == 5
  Manual Failure Mode Selection : Subsystem  TreatAsAtomicUnit=on
  Max_Motor_Torque_Rear_FM4 [Nm] : Constant  Value=60
  Maximum_Force_Longitudinal_Slip [N] : Constant  Value=1364.44
  Merge : Merge
  Merge Tq_RL : Merge  Inputs=4
  Merge Tq_RR : Merge  Inputs=4
  Merge2 : Merge
  Merge3 : Merge  Inputs=3
  Rigid Axle : Subsystem  TreatAsAtomicUnit=on
  Steering TV with TC : Subsystem  TreatAsAtomicUnit=on
  "Steering Wheel Saturation (per site) [deg] " : Constant  Value=10
  Terminator{,1..9} (10 alike) : Terminator
  Transmission_Gear_Ratio_MtoW : Constant  Value=4
  Transmission_Gear_Ratio_WtoM : Constant  Value=1/4
  VDC Complete : Subsystem  TreatAsAtomicUnit=on
  VDC without Longitudinal : Subsystem  TreatAsAtomicUnit=on
  Wheel_Radius [m] : Constant  Value=0.2285
  Tq_RR [Nm] (0,inf) : Outport  VectorParamsAs1DForOutWhenUnconnected=off
  Tq_RL [Nm] (0,inf) : Outport  Port=2  VectorParamsAs1DForOutWhenUnconnected=off
  Tq_RRwc [Nm] (0,inf) : Outport  Port=3  VectorParamsAs1DForOutWhenUnconnected=off
  Tq_RLwc [Nm] (0,inf) : Outport  Port=4  VectorParamsAs1DForOutWhenUnconnected=off
  MaxTq_RR [Nm] (0,inf) : Outport  Port=5  VectorParamsAs1DForOutWhenUnconnected=off
  MaxTq_RL [Nm] (0,inf) : Outport  Port=6  VectorParamsAs1DForOutWhenUnconnected=off
  MaxFx_RR [N] (0,inf) : Outport  Port=7  VectorParamsAs1DForOutWhenUnconnected=off
  MaxFx_RL [N] (0,inf) : Outport  Port=8  VectorParamsAs1DForOutWhenUnconnected=off
  Throttle [0-1] (0-100%) : Outport  Port=9  VectorParamsAs1DForOutWhenUnconnected=off
  Fy_R [N] (0,inf) : Outport  Port=10  VectorParamsAs1DForOutWhenUnconnected=off
  Mass [kg] (0,inf) : Outport  Port=11  VectorParamsAs1DForOutWhenUnconnected=off
  Handling [-] (-inf,inf) : Outport  Port=12  VectorParamsAs1DForOutWhenUnconnected=off
  Flags [num5] : Outport  Port=13  VectorParamsAs1DForOutWhenUnconnected=off
  SKF_act : Outport  Port=14  VectorParamsAs1DForOutWhenUnconnected=off
  CKF_act : Outport  Port=15  VectorParamsAs1DForOutWhenUnconnected=off
  wires:
  VDC Complete/4(Tq_RLwc [Nm] (0,inf)) -> Tq_RLwc [Nm] (0,inf)/1
  VDC Complete/3(Tq_RRwc [Nm] (0,inf)) -> Tq_RRwc [Nm] (0,inf)/1
  VDC Complete/5(MaxTq_RR [Nm] (0,inf)) -> MaxTq_RR [Nm] (0,inf)/1
  VDC Complete/6(MaxTq_RL [Nm] (0,inf)) -> MaxTq_RL [Nm] (0,inf)/1
  VDC Complete/7(MaxFx_RR [N] (0,inf)) -> MaxFx_RR [N] (0,inf)/1
  VDC Complete/8(MaxFx_RL [N] (0,inf)) -> MaxFx_RL [N] (0,inf)/1
  VDC Complete/9(Throttle [0-1] (0-100%)) -> Throttle [0-1] (0-100%)/1
  VDC Complete/10(Fy_R [N] (0,inf)) -> Fy_R [N] (0,inf)/1
  VDC Complete/11(Mass [kg] (0,inf)) -> Mass [kg] (0,inf)/1
  VDC Complete/12(Handling [-] (-inf,inf)) -> Handling [-] (-inf,inf)/1
  VDC without Longitudinal/3(MaxTq_RR [Nm] (0,inf)) -> Terminator/1
  VDC without Longitudinal/4(MaxTq_RL [Nm] (0,inf)) -> Terminator1/1
  VDC without Longitudinal/5(MaxFx_RR [N] (0,inf)) -> Terminator2/1
  VDC without Longitudinal/6(MaxFx_RL [N] (0,inf)) -> Terminator3/1
  VDC without Longitudinal/7(Fy_R [N] (0,inf)) -> Terminator4/1
  VDC without Longitudinal/8(Throttle [0-1] (0-100%)) -> Terminator5/1
  VDC without Longitudinal/9(Mass [kg] (0,inf)) -> Terminator6/1
  VDC without Longitudinal/10(Handling [-] (-inf,inf)) -> Terminator7/1
  VDC without Longitudinal/11(Tq_RRwc [Nm] (0,inf)) -> Terminator8/1
  VDC without Longitudinal/12(Tq_RLwc [Nm] (0,inf)) -> Terminator9/1
  VDC Complete/13(Flags_[num5]) -> Flags [num5]/1
  Merge2/1 -> SKF_act/1
  Merge3/1 -> CKF_act/1
  "Steering Wheel Saturation (per site) [deg] "/1 -> VDC without Longitudinal/5(Steering Saturation (per site) [deg]), VDC Complete/5(Steering Saturation (per site) [deg]), Steering TV with TC/5("Steering Wheel Saturation (per site) ")
  SKF_Initial/1 -> VDC without Longitudinal/6(SKF_initial), VDC Complete/6(SKF_Initial), Steering TV with TC/6(SKF_Initial)
  CKF_Initial/1 -> VDC Complete/7(CKF_Initial), VDC without Longitudinal/7(CKF_Initial), Steering TV with TC/7(CKF_Initial)
  Cte_SKF/1 -> VDC without Longitudinal/8(Cte_SKF), VDC Complete/8(Cte_SKF), Steering TV with TC/8(Cte_SKF)
  Cte_CKF/1 -> VDC without Longitudinal/9(Cte_CKF), VDC Complete/9(Cte_CKF), Steering TV with TC/9(Cte_CKF)
  RL_AngularVel_Motor [rad/s]/1 -> VDC without Longitudinal/10(AngularVelocity_Motor_RL [rad/s]), VDC Complete/10(AngularVelocity_Motor_RL [rad/s]), Steering TV with TC/10(AngVel_RL_Motor)
  RR_AngularVel_Motor [rad/s]/1 -> VDC without Longitudinal/11(AngularVelocity_Motor_RR [rad/s]), VDC Complete/11(AngularVelocity_Motor_RR [rad/s]), Steering TV with TC/11(AngVel_RR_Motor)
  Steering TV with TC/3(SKF_act) -> [SKF_act3]
  Steering TV with TC/4(CKF_act) -> [CKF_act3]
  VDC without Longitudinal/13(CKF_act) -> [CKF_act2]
  VDC Complete/14(SKF_act) -> [SKF_act1]
  VDC Complete/15(CKF_act) -> [CKF_act1]
  [CKF_act2] -> Merge3/2
  [CKF_act1] -> Merge3/1
  [CKF_act3] -> Merge3/3
  [SKF_act1] -> Merge2/1
  [SKF_act3] -> Merge2/2
  FAILURE MODE/1 -> VDC Complete/Action
  FAILURE MODE/2 -> VDC without Longitudinal/Action
  FAILURE MODE/3 -> Steering TV with TC/Action
  FAILURE MODE/4 -> Rigid Axle/Action
  FR_Susp [N]/1 -> VDC without Longitudinal/13(FR_Susp [N]), VDC Complete/13(FR_Susp [N])
  FL_Susp [N]/1 -> VDC Complete/14(FL_Susp [N]), VDC without Longitudinal/14(FL_Susp [N])
  RR_Susp [N]/1 -> VDC Complete/15(RR_Susp [N]), VDC without Longitudinal/15(RR_Susp [N])
  RL_Susp [N]/1 -> VDC Complete/16(RL_Susp [N]), VDC without Longitudinal/16(RL_Susp [N])
  Steering TV with TC/1(Tq_RR_FM3 [Nm] (0,inf)) -> [Tq_RR_FM3]
  Steering TV with TC/2(Tq_RL_FM3 [Nm] (0,inf)) -> [Tq_RL_FM3]
  VDC without Longitudinal/1(Tq_RR_FM2 [Nm] (0,inf)) -> [Tq_RR_FM2]
  VDC Complete/1(Tq_RR_FM1 [Nm] (0,inf)) -> [Tq_RR_FM1]
  VDC Complete/2(Tq_RL_FM1 [Nm] (0,inf)) -> [Tq_RL_FM1]
  Merge Tq_RR/1 -> Tq_RR [Nm] (0,inf)/1
  Rigid Axle/1(Tq_RR_FM4 [Nm] (0,inf)) -> [Tq_RR_FM4]
  Rigid Axle/2(Tq_RL_FM4 [Nm] (0,inf)) -> [Tq_RL_FM4]
  Merge Tq_RL/1 -> Tq_RL [Nm] (0,inf)/1
  [Tq_RR_FM1] -> Merge Tq_RR/4
  [Tq_RR_FM2] -> Merge Tq_RR/3
  [Tq_RR_FM3] -> Merge Tq_RR/2
  [Tq_RR_FM4] -> Merge Tq_RR/1
  [Tq_RL_FM1] -> Merge Tq_RL/4
  [Tq_RL_FM2] -> Merge Tq_RL/3
  [Tq_RL_FM3] -> Merge Tq_RL/2
  [Tq_RL_FM4] -> Merge Tq_RL/1
  Brake Pedal (0-1) [-]/1 -> Steering TV with TC/12(Bp), VDC Complete/19(Brake Pedal (0-1) [-]), VDC without Longitudinal/19(Brake Pedal (0-1) [-])
  Max Regen Torque [Nm]/1 -> VDC Complete/18(Max Regen Torque [Nm]), VDC without Longitudinal/18(Max Regen Torque [Nm]), Steering TV with TC/13(Max_Regen_Tq)
  Regenerative Enable [0,1]/1 -> VDC Complete/17(Regenerative Enable [0,1]), VDC without Longitudinal/17(Regenerative Enable [0,1]), Steering TV with TC/14(Regen_enable)
  If/1 -> Automatic Failure Mode/Action
  FAILURE_MODE/1 -> Automatic Failure Mode/1(In1)
  If/2 -> Manual Failure Mode Selection/Action
  Constant/1 -> [FM_select], If/1
  [FM_select] -> Manual Failure Mode Selection/1(In1)
  Merge/1 -> FAILURE MODE/1
  Automatic Failure Mode/1(Out1) -> Merge/1
  Manual Failure Mode Selection/1(Out1) -> Merge/2
  VDC without Longitudinal/2(Tq_RL_FM2 [Nm] (0,inf)) -> [Tq_RL_FM2]
  [Ellipse_Accel_X_Y_Z] -> VDC without Longitudinal/12(Ellipse_acc_ax_ay_az)
  [Ellipse_Accel_X_Y_Z] -> VDC Complete/12(Ellipse_acc)
  [Ellipse_Gyro_X_Y_Z] -> VDC Complete/20(Gyro_Ellipse)
  [Ellipse_Vel_X_Y_Z] -> VDC Complete/21(Ellipse_vel)
  Gas Pedal (0-1) [-]/1 -> [gas_pedal_0_1]
  [gas_pedal_0_1] -> Rigid Axle/3(Gas Pedal [0-1])
  [gas_pedal_0_1] -> Steering TV with TC/3(Gas Pedal [0-1])
  [gas_pedal_0_1] -> VDC without Longitudinal/3(Gas Pedal (0-1) [-])
  [gas_pedal_0_1] -> VDC Complete/3(Gas Pedal (0-1) [-])
  Ap_Sat_Up/1 -> [ap_sat_up]
  Ap_Sat_Down/1 -> [ap_sat_down]
  [ap_sat_up] -> Rigid Axle/1("Ap_Sat_up ")
  [ap_sat_down] -> Rigid Axle/2(Ap_Sat_down)
  [ap_sat_up] -> Steering TV with TC/1("Ap_Sat_up ")
  [ap_sat_down] -> Steering TV with TC/2(Ap_Sat_down)
  [ap_sat_up] -> VDC without Longitudinal/1(Ap_Sat_Up [-])
  [ap_sat_down] -> VDC without Longitudinal/2(Ap_Sat_Down [-])
  [ap_sat_down] -> VDC Complete/2(Ap_Sat_Down [-])
  [ap_sat_up] -> VDC Complete/1(Ap_Sat_Up [-])
  Steering_Angle [deg]/1 -> Gain/1
  Gain/1 -> [steering_angle_normalized]
  [steering_angle_normalized] -> Steering TV with TC/4(Steering_Angle [deg])
  [steering_angle_normalized] -> VDC without Longitudinal/4(Steering_Angle [deg])
  [steering_angle_normalized] -> VDC Complete/4(Steering_Angle [deg])
  Max_Motor_Torque_Rear_FM4 [Nm]/1 -> [Max_Motor_Torque_Rear_FM4]
  [Max_Motor_Torque_Rear_FM4] -> Rigid Axle/4(Max_Motor_Torque_Rear_FM4 [Nm])
  Transmission_Gear_Ratio_MtoW/1 -> [Gear_Ratio_MtoW]
  [Gear_Ratio_MtoW] -> Rigid Axle/5(Gear_Ratio_MtoW)
  [Ellipse_Vel_X_Y_Z] -> Steering TV with TC/15(Ellipse_Vel (x,y,z))
  Wheel_Radius [m]/1 -> [Wheel_Radius]
  Transmission_Gear_Ratio_WtoM/1 -> [Gear_Ratio_WtoM]
  Maximum_Force_Longitudinal_Slip [N]/1 -> [Max_Wheel_Fx]
  Ellipse_Euler(roll,pitch,yaw) [rad]/1 -> [Ellipse_EulerAngles]
  Ellipse_Accel(ax,ay,az) [m/s2]/1 -> [Ellipse_Accel_X_Y_Z]
  Ellipse_Vel(vx,vy,vz) [m/s]/1 -> [Ellipse_Vel_X_Y_Z]
  Ellipse_Gyro(gx,gy,gz) [rad/s]/1 -> [Ellipse_Gyro_X_Y_Z]

== system Torque_Control/VDC/WORKSHOP_MODE_RESTRICTIONS ==
  Workshop_Mode_Enable : Inport
  Torque_R_in : Inport  Port=2
  Torque_L_in : Inport  Port=3
  BYPASS : Subsystem  TreatAsAtomicUnit=on
  If : If  IfExpression=u1 == 1
  Merge : Merge
  Merge1 : Merge
  Saturation : Saturate  UpperLimit=580  LowerLimit=-580
  Saturation1 : Saturate  UpperLimit=580  LowerLimit=-580
  "Torque_Reduction " : Subsystem  TreatAsAtomicUnit=on
  Torque_L_out : Outport  VectorParamsAs1DForOutWhenUnconnected=off
  Torque_R_out : Outport  Port=2  VectorParamsAs1DForOutWhenUnconnected=off
  wires:
  If/2 -> BYPASS/Action
  If/1 -> "Torque_Reduction "/Action
  Workshop_Mode_Enable/1 -> If/1
  Torque_R_in/1 -> "Torque_Reduction "/1(In1), BYPASS/1(In1)
  Torque_L_in/1 -> "Torque_Reduction "/2(In2), BYPASS/2(In2)
  BYPASS/1(Out1) -> Merge/1
  BYPASS/2(Out2) -> Merge1/2
  "Torque_Reduction "/1(Out1) -> Merge/2
  "Torque_Reduction "/2(Out2) -> Merge1/1
  Merge/1 -> Saturation/1
  Merge1/1 -> Saturation1/1
  Saturation/1 -> Torque_R_out/1
  Saturation1/1 -> Torque_L_out/1

== system Torque_Control/Accumulator Power/PowerLimitDetection/LimitReached ==
  Action Port : ActionPort  ActionPortLabel=if { }
  Constant : Constant
  "Out " : Outport  VectorParamsAs1DForOutWhenUnconnected=off
  wires:
  Constant/1 -> "Out "/1

== system Torque_Control/Accumulator Power/PowerLimitDetection/OK_OrLatch ==
  IN : Inport
  Action Port : ActionPort  ActionPortLabel=else { }
  If : If  IfExpression=(u1>0)
  Latched Error : Subsystem  TreatAsAtomicUnit=on
  Merge : Merge
  OK : Subsystem  TreatAsAtomicUnit=on
  Out 1 : Outport  VectorParamsAs1DForOutWhenUnconnected=off
  wires:
  IN/1 -> If/1
  If/1 -> Latched Error/Action
  If/2 -> OK/Action
  Latched Error/1("Out ") -> Merge/1
  OK/1("Out ") -> Merge/2
  Merge/1 -> Out 1/1

== system Torque_Control/Power Limitation Temperature/temperature_SoP/temperature_rise_limitator_Accu ==
  note: initial_limitation es una constante para la reducción inicial (de 0 a 1, más bajo significa que cambia
      | menos, más alto la limitación
      | inicial es más bestia).
  note: saturamos de 1 a 0 por si acaso
  note: magia chunga para
      | que los números cuadren
  note: Se limita la corriente en proporción
      | al ratio entre la temperatura actual y 50ºC
  note: output 0 si está por
      | debajo de 50ºC, 1 si está
      | por encima
  max_cell_temp : Inport
  initial_limitation : Inport  Port=2
  Add1 : Sum  Inputs=-+
  Add2 : Sum  Inputs=-++
  Add3 : Sum  Inputs=+-
  Constant1 : Constant  Value=45
  Constant2 : Constant  Value=5
  Constant3 : Constant
  Divide : Product  Inputs=*/
  Low-Pass Filter (Discrete or Continuous)1 : eeGeneralControl/Low-Pass Filter (Discrete or Continuous)  K=1  T=100  B=inf  A=-inf  init_option=Inherited from block input  x0=0  Ts=-1
  Product4 : Product
  Saturation1 : Saturate  UpperLimit=1  LowerLimit=0
  Temp higher than 50 : simulink/Logic and Bit Operations/Compare To Constant  relop=>=  const=50  OutDataTypeStr=boolean  ZeroCross=off
  SoP : Outport
  wires:
  Divide/1 -> Add3/1
  Constant3/1 -> Add2/3
  Constant1/1 -> Divide/1
  max_cell_temp/1 -> Add1/2, Temp higher than 50/1
  Temp higher than 50/1 -> Add2/1, Product4/2
  Constant2/1 -> Add1/1
  Product4/1 -> Add2/2
  Add2/1 -> Low-Pass Filter (Discrete or Continuous)1/1
  Add3/1 -> Product4/1
  Add1/1 -> Divide/2
  Saturation1/1 -> SoP/1
  initial_limitation/1 -> Add3/2
  Low-Pass Filter (Discrete or Continuous)1/1 -> Saturation1/1

== system Torque_Control/Power Limitation Temperature/temperature_SoP/temperature_rise_limitator_Inverters ==
  note: output 0 si está por
      | debajo de 50ºC, 1 si está
      | por encima
  note: Se limita la corriente en proporción
      | al ratio entre la temperatura actual y 50ºC
  note: magia chunga para
      | que los números cuadren
  note: saturamos de 1 a 0 por si acaso
  note: initial_limitation es una constante para la reducción inicial (de 0 a 1, más bajo significa que cambia
      | menos, más alto la limitación
      | inicial es más bestia).
  max_inverter_temp : Inport
  initial_limitation : Inport  Port=2
  Add1 : Sum  Inputs=-+
  Add2 : Sum  Inputs=-++
  Add3 : Sum  Inputs=+-
  Constant1 : Constant  Value=45
  Constant2 : Constant  Value=5
  Constant3 : Constant
  Divide : Product  Inputs=*/
  Low-Pass Filter (Discrete or Continuous) : eeGeneralControl/Low-Pass Filter (Discrete or Continuous)  K=1  T=100  B=inf  A=-inf  init_option=Inherited from block input  x0=0  Ts=-1
  Product4 : Product
  Saturation1 : Saturate  UpperLimit=1  LowerLimit=0
  Temp higher than 50 : simulink/Logic and Bit Operations/Compare To Constant  relop=>=  const=50  OutDataTypeStr=boolean  ZeroCross=off
  SoP : Outport
  wires:
  Low-Pass Filter (Discrete or Continuous)/1 -> Saturation1/1
  initial_limitation/1 -> Add3/2
  Saturation1/1 -> SoP/1
  Add1/1 -> Divide/2
  Add3/1 -> Product4/1
  Add2/1 -> Low-Pass Filter (Discrete or Continuous)/1
  Product4/1 -> Add2/2
  Constant2/1 -> Add1/1
  Temp higher than 50/1 -> Product4/2, Add2/1
  max_inverter_temp/1 -> Temp higher than 50/1, Add1/2
  Constant1/1 -> Divide/1
  Constant3/1 -> Add2/3
  Divide/1 -> Add3/1
